simulink model "rlc"  (R2020b)
settings: Solver=FixedStepAuto  StartTime=0.0  StopTime=Tk  FixedStep=Ts  RelTol=1e-3
undefined symbols (not defined in the file or in its folder): C, L, R, Ts
settings Model: Creator=Rampage  LastModifiedBy=Rampage

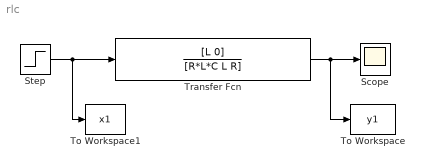
== system rlc ==
  Scope : Scope
  Step : Step  Time=Ts  Before=1  After=0  SampleTime=0
  To Workspace : ToWorkspace  VariableName=y1  SampleTime=-1
  To Workspace1 : ToWorkspace  VariableName=x1  SampleTime=-1
  Transfer Fcn : TransferFcn  Numerator=[L 0]  Denominator=[R*L*C L R]
  wires:
  Step/1 -> To Workspace1/1, Transfer Fcn/1
  Transfer Fcn/1 -> Scope/1, To Workspace/1
